simulink model "mdlmalthus"  (Simulink 7.8)
settings: Solver=ode45  StartTime=0.0  StopTime=10.0  RelTol=1e-3
settings Model: Creator=marekpesta  LastModifiedBy=polacekm

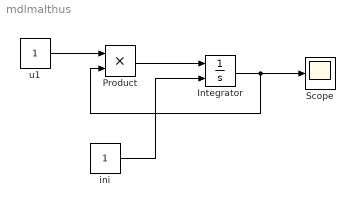
== system mdlmalthus ==
  Integrator : Integrator  InitialConditionSource=external
  Product : Product  RndMeth=Zero
  Scope : Scope
      settings: SaveName=sc
  ini : Constant
  u1 : Constant
  wires:
  u1/1 -> Product/1
  Product/1 -> Integrator/1
  ini/1 -> Integrator/2
  Integrator/1 -> Product/2, Scope/1
